simulink model "Verifica_LQR_11032026"  (R2025b)
settings: Solver=VariableStepAuto  StartTime=0.0  StopTime=50.0  RelTol=1e-3
values from neighbouring files (symbols this model uses):
  A = double(subs(A_sym, x, x_star))    [SvolgimentoEsame_11032026.m]
  B = double(subs(B_sym, x, x_star))    [SvolgimentoEsame_11032026.m]
  q1_ref = 0.5    [SvolgimentoEsame_11032026.m]
undefined symbols (not defined in the file or in its folder): D_tot, K_LQR_i, K_LQR_x, n
settings Model: Creator=salvo  LastModifiedBy=salvo

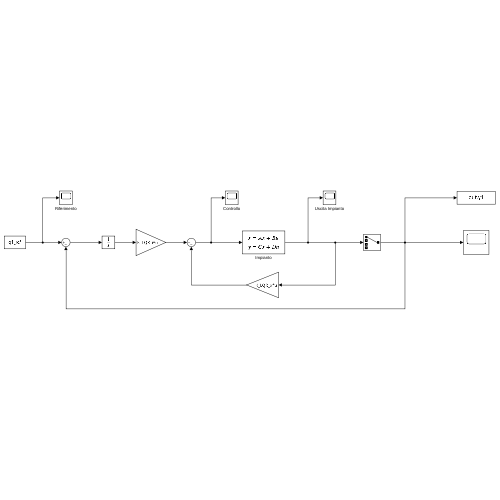
[thumbnail: Simulink's stored preview of the top-level diagram]
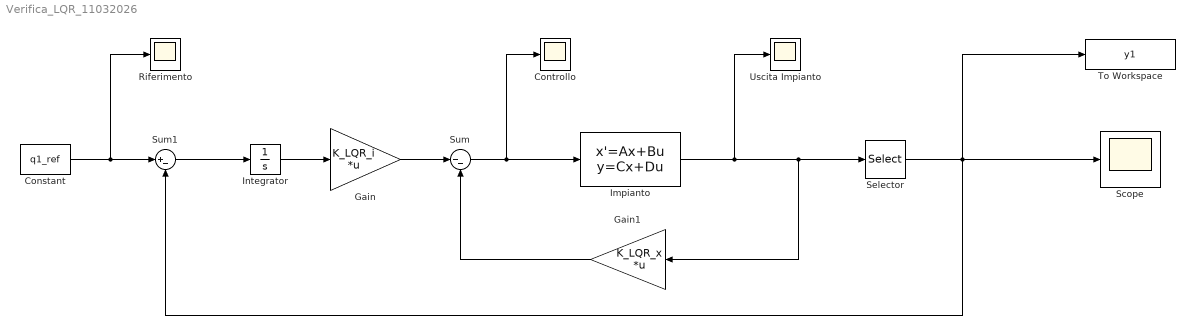
== system Verifica_LQR_11032026 ==
  Constant : Constant  Value=q1_ref
  Controllo : Scope
      settings: ActiveDisplayYMinimum=-3.4803944007461247  ActiveDisplayYMaximum=17.095004597613659  DataLoggingVariableName=ScopeData2
  Gain : Gain  Gain=K_LQR_i  Multiplication=Matrix(K*u)
  Gain1 : Gain  Gain=K_LQR_x  Multiplication=Matrix(K*u)
  Impianto : StateSpace  A=A  B=B  C=eye(n)  D=D_tot  InitialCondition=0
  Integrator : Integrator
  Riferimento : Scope
      settings: ActiveDisplayYMinimum=0.4  ActiveDisplayYMaximum=0.6
  Scope : Scope
      settings: ActiveDisplayYMinimum=0.11332274326091707  ActiveDisplayYMaximum=0.837135894209821
  Selector : Selector  InputPortWidth=4  IndexOptions=Index vector (dialog)  Indices=1  OutputSizes=1
  Sum : Sum  Inputs=|--
  Sum1 : Sum  Inputs=|+-
  To Workspace : ToWorkspace  VariableName=y1  SaveFormat=Timeseries  SampleTime=-1
  Uscita Impianto : Scope
      settings: ActiveDisplayYMinimum=-0.14310149064248157  ActiveDisplayYMaximum=0.69643263559808566  DataLoggingVariableName=ScopeData3
  wires:
  Constant/1 -> Riferimento/1, Sum1/1
  Impianto/1 -> Uscita Impianto/1, Gain1/1, Selector/1
  Gain1/1 -> Sum/2
  Sum/1 -> Controllo/1, Impianto/1
  Gain/1 -> Sum/1
  Integrator/1 -> Gain/1
  Sum1/1 -> Integrator/1
  Selector/1 -> Sum1/2, To Workspace/1, Scope/1
